simulink model "plant_th"  (R2020a)
settings: Solver=VariableStepAuto  StartTime=0.0  StopTime=simTime  RelTol=1e-3
values from neighbouring files (symbols this model uses):
  flowSpeed = 10    [plant_ts.m]
  rollAng = 30*pi/180    (= 0.523598775598)    [plant_ts.m]
libraries: plant x1
settings Model: Creator=Ayaz  LastModifiedBy=Ayaz

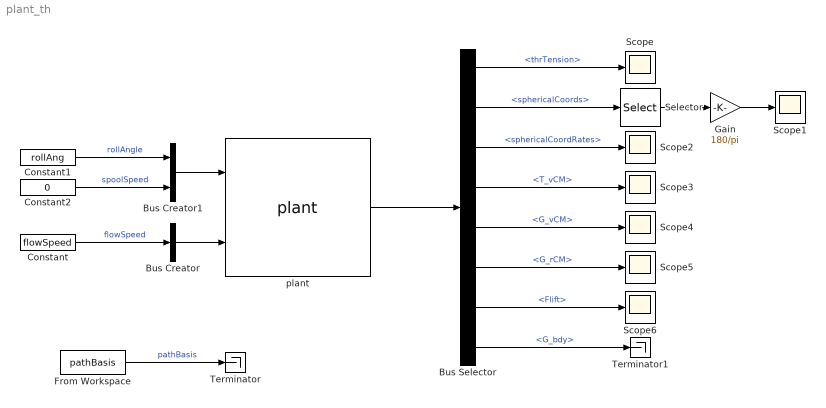
== system plant_th ==
  Bus Creator : BusCreator  Inputs=1
  Bus Creator1 : BusCreator  Inputs=2
  Bus Selector : BusSelector  OutputSignals=thrTension,sphericalCoords,sphericalCoordRates,T_vCM,G_vCM,G_rCM,Flift,G_bdy
  Constant : Constant  Value=flowSpeed
  Constant1 : Constant  Value=rollAng
  Constant2 : Constant  Value=0
  From Workspace : FromWorkspace  VariableName=pathBasis
  Gain : Gain  Gain=180/pi
  Scope{,1..6} (7 alike) : Scope
  Selector : Selector  InputPortWidth=3  IndexOptions=Index vector (dialog)  Indices=[1 2]  OutputSizes=1
  Terminator : Terminator
  Terminator1 : Terminator
  plant : plant/plant  AoA=AoA  init_radius=init_R  init_azim=init_azim  init_elev=init_elev  init_dAzim=init_azimRate  init_dElev=init_elevRate  gravEnable=on  fluidEnable=on  mass=kiteMass  refArea=refArea  aeroCent=aeroCent  AoA_vals=AoA_vals  CL_vals=CL_vals  CD_vals=CD_vals  flowDensity=rho  gravAccel=gravAccl
  wires:
  Constant/1 -> Bus Creator/1  "flowSpeed"
  Bus Creator/1 -> plant/2
  Bus Creator1/1 -> plant/1
  Constant1/1 -> Bus Creator1/1  "rollAngle"
  Constant2/1 -> Bus Creator1/2  "spoolSpeed"
  plant/1 -> Bus Selector/1
  Bus Selector/1 -> Scope/1  "<thrTension>"
  Bus Selector/3 -> Scope2/1  "<sphericalCoordRates>"
  Bus Selector/4 -> Scope3/1  "<T_vCM>"
  Bus Selector/5 -> Scope4/1  "<G_vCM>"
  Bus Selector/6 -> Scope5/1  "<G_rCM>"
  Bus Selector/7 -> Scope6/1  "<Flift>"
  From Workspace/1 -> Terminator/1  "pathBasis"
  Bus Selector/2 -> Selector/1  "<sphericalCoords>"
  Selector/1 -> Gain/1
  Gain/1 -> Scope1/1
  Bus Selector/8 -> Terminator1/1  "<G_bdy>"
